simulink library "Lib_Mask"  (R2025b)
settings: Solver=VariableStepAuto  StartTime=0.0  StopTime=10.0  RelTol=1e-3
settings Model: Creator=soura  LastModifiedBy=soura
settings RTWCC: GPUComputeCapability=3.5

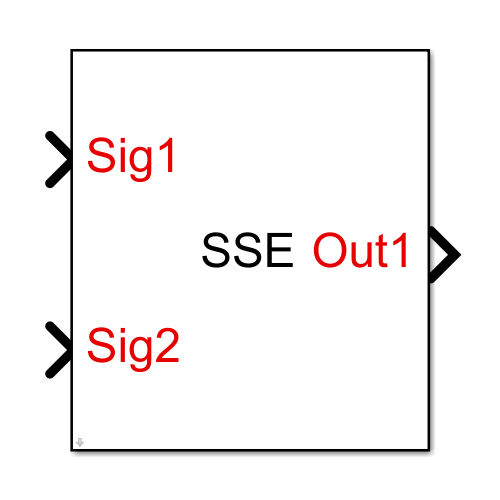
[thumbnail: Simulink's stored preview of the top-level diagram]
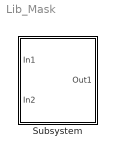
== system Lib_Mask ==
  Subsystem : Subsystem  mask{scale=1}
      mask DialogControl Control Prompt: Enter the Scaling factor
      mask Display:
      | disp('SSE');
      | color('red');
      | port_label('Input', 2, 'Sig2');
      | port_label('Input',1,'Sig1')
      | port_label('output', 1, 'Out1');

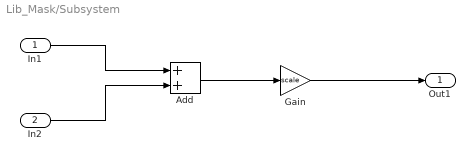
== system Lib_Mask/Subsystem ==
  In1 : Inport
  In2 : Inport  Port=2
  Add : Sum
  Gain : Gain  Gain=scale
  Out1 : Outport
  wires:
  Add/1 -> Gain/1
  In1/1 -> Add/1
  In2/1 -> Add/2
  Gain/1 -> Out1/1
